simulink model "myModel3"  (R2018b)
settings: Solver=VariableStepAuto  StartTime=0.0  StopTime=4  RelTol=1e-3
libraries: simulink x1
settings Model: Creator=lorenzo  LastModifiedBy=lorenzo

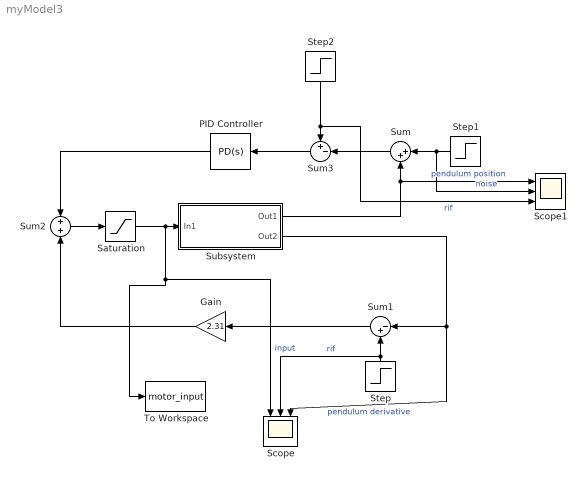
== system myModel3 ==
  Gain : Gain  Gain=2.31
  PID Controller : simulink/Continuous/PID Controller  Controller=PD  Form=Parallel  TimeDomain=Continuous-time  SampleTime=-1  IntegratorMethod=Forward Euler  FilterMethod=Forward Euler  ControllerParametersSource=internal  P=21.3  I=1  D=4.473  UseFilter=on  N=1000  TunerSelectOption=Frequency Response Based  InitialConditionSource=internal  InitialConditionForIntegrator=0  InitialConditionForFilter=0  DifferentiatorICPrevScaledInput=0  ExternalReset=none  TrackingMode=off  Kt=1  LimitOutput=off  UpperSaturationLimit=inf  LowerSaturationLimit=-inf  LinearizeAsGain=on  AntiWindupMode=none  Kb=1  POutMin=[]  POutMax=[]  IOutMin=[]  IOutMax=[]  DOutMin=[]  DOutMax=[]  NOutMin=[]  NOutMax=[]  SumOutMin=[]  SumOutMax=[]  SaturationOutMin=[]  SaturationOutMax=[]  PParamMin=[]  PParamMax=[]  IParamMin=[]  IParamMax=[]  DParamMin=[]  DParamMax=[]  NParamMin=[]  NParamMax=[]  KbParamMin=[]  KbParamMax=[]  KtParamMin=[]  KtParamMax=[]  KbOutMin=[]  KbOutMax=[]  KtOutMin=[]  KtOutMax=[]  IntegratorOutMin=[]  IntegratorOutMax=[]  FilterOutMin=[]  FilterOutMax=[]  SumI1OutMin=[]  SumI1OutMax=[]  SumI2OutMin=[]  SumI2OutMax=[]  SumI3OutMin=[]  SumI3OutMax=[]  SumI4OutMin=[]  SumI4OutMax=[]  SumDOutMin=[]  SumDOutMax=[]  DifferentiatorOutMin=[]  DifferentiatorOutMax=[]  FilterDiffOutCoefMin=[]  FilterDiffOutCoefMax=[]  ReciprocalOutMin=[]  ReciprocalOutMax=[]  SumDenOutMin=[]  SumDenOutMax=[]  SumNumOutMin=[]  SumNumOutMax=[]  DivideOutMin=[]  DivideOutMax=[]  IntegratorContinuousStateAttributes=''  IntegratorStateMustResolveToSignalObject=off  IntegratorRTWStateStorageClass=Auto  FilterContinuousStateAttributes=''  FilterStateMustResolveToSignalObject=off  FilterRTWStateStorageClass=Auto  ParallelPVariant=InternalParameters  IdealPVariant=Disabled  IVariant=Disabled  DVariant=InternalParameters  IntegratorVariant=Disabled  SatVariant=Disabled  AWVariant=Disabled  PCopyVariant=Disabled  TRVariant=Disabled  FdbkBlocksVariant=Forward  IdealPFdbkVariant=Disabled  SatFdbkVariant=Disabled  DerivativeFilterVariant=ContFilter  NVariant=InternalParameters  NCopyVariant=Disabled  FilterICVariant=InternalICsFilter  IntegratorICVariant=Disabled  ExternalResetVariant=Disabled  TRSumVariant=Passthrough  SumFdbkVariant=Disabled  SumVariant=Sum_PD
  Saturation : Saturate  UpperLimit=10  LowerLimit=-10
  Scope : Scope  NumInputPorts=3
  Scope1 : Scope  NumInputPorts=3
  Step : Step  Time=2.5  After=2.5  SampleTime=0
  Step1 : Step  Time=1.5  After=0.2  SampleTime=0
  Step2 : Step  After=0  SampleTime=0
  Subsystem : Subsystem
  Sum : Sum  Inputs=|++
  Sum1 : Sum  Inputs=|-+
  Sum2 : Sum  Inputs=+|+
  Sum3 : Sum  Inputs=+-|
  To Workspace : ToWorkspace  VariableName=motor_input  SaveFormat=Timeseries  SampleTime=-1
  wires:
  Subsystem/1(Out1) -> Sum/2, Scope1/1  "pendulum position"
  Step1/1 -> Scope1/2, Sum/1  "noise"
  Step/1 -> Scope/2, Sum1/2  "rif"
  Step2/1 -> Scope1/3, Sum3/1  "rif"
  Sum/1 -> Sum3/2
  Sum2/1 -> Saturation/1
  Subsystem/2(Out2) -> Scope/3, Sum1/1  "pendulum derivative"
  Sum1/1 -> Gain/1
  Sum3/1 -> PID Controller/1
  PID Controller/1 -> Sum2/1
  Gain/1 -> Sum2/2
  Saturation/1 -> To Workspace/1, Scope/1, Subsystem/1(In1)  "input"

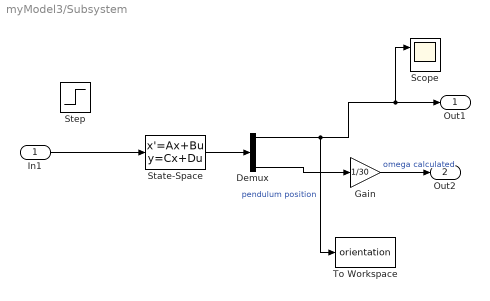
== system myModel3/Subsystem ==
  In1 : Inport
  Demux : Demux
  Gain : Gain  Gain=1/30
  Scope : Scope  NumInputPorts=2
  State-Space : StateSpace  A=[0 1 0; 23.5031 0 0.0045; -23.5031 0 -19.9513]  B=[0; 0.1393; -621.6819]  C=[107.47 0 0; 1 0 0; 0 1 0; 0 0 1]  D=[0; 0; 0; 0]  InitialCondition=[0.2/107.47;0;0]
  Step : Step  SampleTime=0
  To Workspace : ToWorkspace  VariableName=orientation  SaveFormat=Timeseries  SampleTime=-1
  Out1 : Outport
  Out2 : Outport  Port=2
  wires:
  State-Space/1 -> Demux/1
  In1/1 -> State-Space/1
  Gain/1 -> Out2/1  "omega calculated"
  Demux/4 -> Gain/1
  Demux/1 -> To Workspace/1, Scope/1, Out1/1  "pendulum position"
